simulink subsystem "Input"  (R2024b)
settings: Solver=VariableStepAuto  StartTime=0.0  StopTime=10.0  RelTol=1e-3
libraries: c2802xlib x9
settings Model: Creator=sgade  LastModifiedBy=sgade

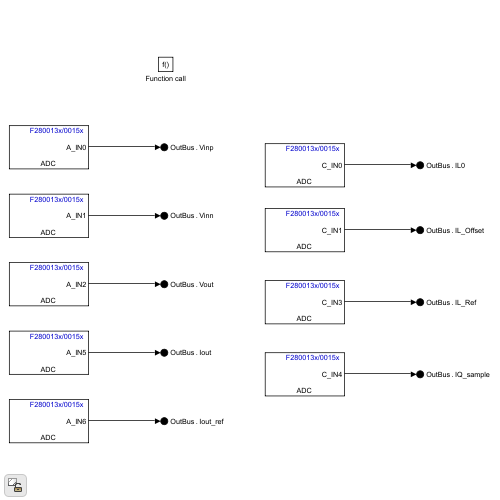
[thumbnail: Simulink's stored preview of the top-level diagram]
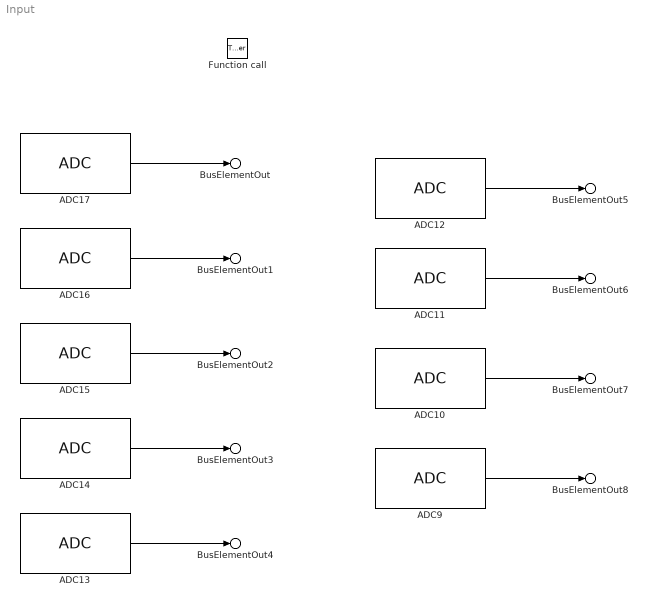
== system Input ==
  Function call : TriggerPort  TriggerType=function-call  VariantControl=(inherit)  PortDimensions=1
  ADC10 : c2802xlib/ADC  blkParamProc=C2000_Type5_001x  ADCModule=C  samplingMode=Single sample mode  ADCResolution=12-bit (Single-ended input)  useSOC1=SOC3  useSOC2=SOC0_SOC1  SOCAcquisitionWindow=8  SOCTriggerSource=ePWM1_ADCSOCA  SOCInterruptTrigger=No ADCINT  Ts=-1  dType=single  postInterrupt=off  interruptSel=ADCINT1  ADCINTContinuous=on  endma=off  chdma=1  conv1=ADCINA0  conv2=ADCINA0 and ADCINB0  conv1_Type4=ADCIN3  conv2_Type4=ADCIN0 and ADCIN1
      settings: LibrarySourceBlock=c280013xlib/ADC
  ADC11 : c2802xlib/ADC  blkParamProc=C2000_Type5_001x  ADCModule=C  samplingMode=Single sample mode  ADCResolution=12-bit (Single-ended input)  useSOC1=SOC1  useSOC2=SOC0_SOC1  SOCAcquisitionWindow=8  SOCTriggerSource=ePWM1_ADCSOCA  SOCInterruptTrigger=No ADCINT  Ts=-1  dType=single  postInterrupt=off  interruptSel=ADCINT1  ADCINTContinuous=on  endma=off  chdma=1  conv1=ADCINA0  conv2=ADCINA0 and ADCINB0  conv1_Type4=ADCIN1  conv2_Type4=ADCIN0 and ADCIN1
      settings: LibrarySourceBlock=c280013xlib/ADC
  ADC12 : c2802xlib/ADC  blkParamProc=C2000_Type5_001x  ADCModule=C  samplingMode=Single sample mode  ADCResolution=12-bit (Single-ended input)  useSOC1=SOC0  useSOC2=SOC0_SOC1  SOCAcquisitionWindow=8  SOCTriggerSource=ePWM1_ADCSOCA  SOCInterruptTrigger=No ADCINT  Ts=-1  dType=single  postInterrupt=off  interruptSel=ADCINT1  ADCINTContinuous=on  endma=off  chdma=1  conv1=ADCINA0  conv2=ADCINA0 and ADCINB0  conv1_Type4=ADCIN0  conv2_Type4=ADCIN0 and ADCIN1
      settings: LibrarySourceBlock=c280013xlib/ADC
  ADC13 : c2802xlib/ADC  blkParamProc=C2000_Type5_001x  ADCModule=A  samplingMode=Single sample mode  ADCResolution=12-bit (Single-ended input)  useSOC1=SOC4  useSOC2=SOC0_SOC1  SOCAcquisitionWindow=8  SOCTriggerSource=ePWM1_ADCSOCA  SOCInterruptTrigger=No ADCINT  Ts=-1  dType=single  postInterrupt=off  interruptSel=ADCINT1  ADCINTContinuous=on  endma=off  chdma=1  conv1=ADCINA0  conv2=ADCINA0 and ADCINB0  conv1_Type4=ADCIN6  conv2_Type4=ADCIN0 and ADCIN1
      settings: LibrarySourceBlock=c280013xlib/ADC
  ADC14 : c2802xlib/ADC  blkParamProc=C2000_Type5_001x  ADCModule=A  samplingMode=Single sample mode  ADCResolution=12-bit (Single-ended input)  useSOC1=SOC3  useSOC2=SOC0_SOC1  SOCAcquisitionWindow=8  SOCTriggerSource=ePWM1_ADCSOCA  SOCInterruptTrigger=No ADCINT  Ts=-1  dType=single  postInterrupt=off  interruptSel=ADCINT1  ADCINTContinuous=on  endma=off  chdma=1  conv1=ADCINA0  conv2=ADCINA0 and ADCINB0  conv1_Type4=ADCIN5  conv2_Type4=ADCIN0 and ADCIN1
      settings: LibrarySourceBlock=c280013xlib/ADC
  ADC15 : c2802xlib/ADC  blkParamProc=C2000_Type5_001x  ADCModule=A  samplingMode=Single sample mode  ADCResolution=12-bit (Single-ended input)  useSOC1=SOC2  useSOC2=SOC0_SOC1  SOCAcquisitionWindow=8  SOCTriggerSource=ePWM1_ADCSOCA  SOCInterruptTrigger=No ADCINT  Ts=-1  dType=single  postInterrupt=off  interruptSel=ADCINT1  ADCINTContinuous=on  endma=off  chdma=1  conv1=ADCINA0  conv2=ADCINA0 and ADCINB0  conv1_Type4=ADCIN2  conv2_Type4=ADCIN0 and ADCIN1
      settings: LibrarySourceBlock=c280013xlib/ADC
  ADC16 : c2802xlib/ADC  blkParamProc=C2000_Type5_001x  ADCModule=A  samplingMode=Single sample mode  ADCResolution=12-bit (Single-ended input)  useSOC1=SOC1  useSOC2=SOC0_SOC1  SOCAcquisitionWindow=8  SOCTriggerSource=ePWM1_ADCSOCA  SOCInterruptTrigger=No ADCINT  Ts=-1  dType=single  postInterrupt=off  interruptSel=ADCINT1  ADCINTContinuous=on  endma=off  chdma=1  conv1=ADCINA0  conv2=ADCINA0 and ADCINB0  conv1_Type4=ADCIN1  conv2_Type4=ADCIN0 and ADCIN1
      settings: LibrarySourceBlock=c280013xlib/ADC
  ADC17 : c2802xlib/ADC  blkParamProc=C2000_Type5_001x  ADCModule=A  samplingMode=Single sample mode  ADCResolution=12-bit (Single-ended input)  useSOC1=SOC0  useSOC2=SOC0_SOC1  SOCAcquisitionWindow=8  SOCTriggerSource=ePWM1_ADCSOCA  SOCInterruptTrigger=No ADCINT  Ts=-1  dType=single  postInterrupt=off  interruptSel=ADCINT1  ADCINTContinuous=on  endma=off  chdma=1  conv1=ADCINA0  conv2=ADCINA0 and ADCINB0  conv1_Type4=ADCIN0  conv2_Type4=ADCIN0 and ADCIN1
      settings: LibrarySourceBlock=c280013xlib/ADC
  ADC9 : c2802xlib/ADC  blkParamProc=C2000_Type5_001x  ADCModule=C  samplingMode=Single sample mode  ADCResolution=12-bit (Single-ended input)  useSOC1=SOC4  useSOC2=SOC0_SOC1  SOCAcquisitionWindow=8  SOCTriggerSource=ePWM1_ADCSOCA  SOCInterruptTrigger=No ADCINT  Ts=-1  dType=single  postInterrupt=on  interruptSel=ADCINT1  ADCINTContinuous=on  endma=off  chdma=1  conv1=ADCINA0  conv2=ADCINA0 and ADCINB0  conv1_Type4=ADCIN4  conv2_Type4=ADCIN0 and ADCIN1
      settings: LibrarySourceBlock=c280013xlib/ADC
  BusElementOut : Outport  Description=ADCA0  PortName=OutBus  Element=Vinp
  BusElementOut1 : Outport  Description=ADCA1  PortName=OutBus  Element=Vinn
  BusElementOut2 : Outport  Description=ADCA2  PortName=OutBus  Element=Vout
  BusElementOut3 : Outport  Description=ADCA5  PortName=OutBus  Element=Iout
  BusElementOut4 : Outport  Description=ADCA6  PortName=OutBus  Element=Iout_ref
  BusElementOut5 : Outport  Description=ADCC0  PortName=OutBus  Element=IL0
  BusElementOut6 : Outport  Description=ADCC1  PortName=OutBus  Element=IL_Offset
  BusElementOut7 : Outport  Description=ADCC3  PortName=OutBus  Element=IL_Ref
  BusElementOut8 : Outport  Description=ADCC4  PortName=OutBus  Element=IQ_sample
  wires:
  ADC9/1 -> BusElementOut8/1
  ADC10/1 -> BusElementOut7/1
  ADC12/1 -> BusElementOut5/1
  ADC16/1 -> BusElementOut1/1
  ADC15/1 -> BusElementOut2/1
  ADC13/1 -> BusElementOut4/1
  ADC14/1 -> BusElementOut3/1
  ADC17/1 -> BusElementOut/1
  ADC11/1 -> BusElementOut6/1
